simulink model "FSFB_PID_Controller"  (R2022a)
settings: Solver=VariableStepAuto  StartTime=0.0  StopTime=10.0  RelTol=1e-3
undefined symbols (not defined in the file): K1, K2, x_0
libraries: dspsigops x1
settings Model: Creator=domin  LastModifiedBy=domin
settings DataIOCC: SaveOutput=off  SaveTime=off
settings DebuggingCC: ModelReferenceExtraNoncontSigs=warning
settings GRTTargetCC: CombineOutputUpdateFcns=off  MatFileLogging=off

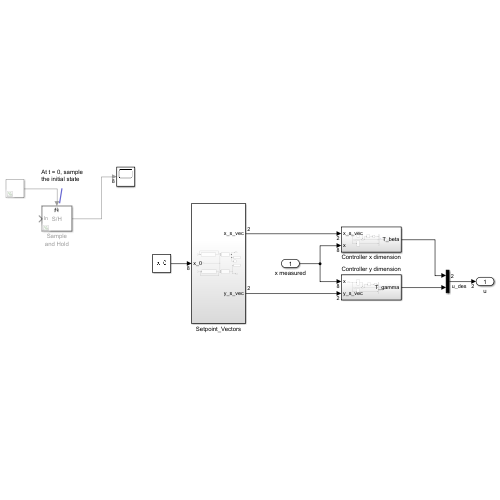
[thumbnail: Simulink's stored preview of the top-level diagram]
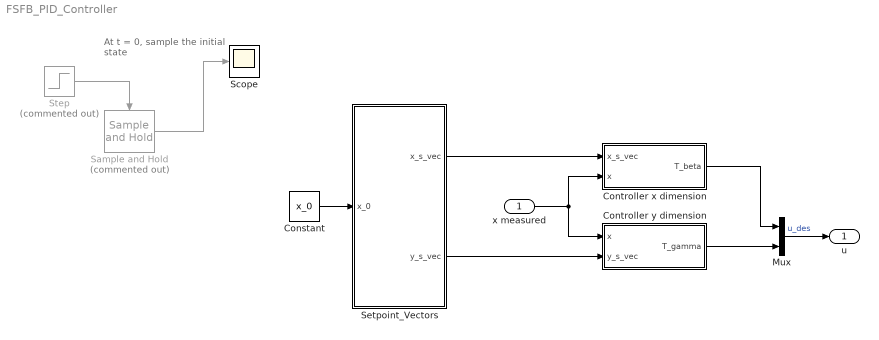
== system FSFB_PID_Controller ==
  note: At t = 0, sample the initial state
  x measured : Inport
  Constant : Constant  Value=x_0
  Controller x dimension : Subsystem
  Controller y dimension : Subsystem
  Mux : Mux  Inputs=2
  Sample and Hold : dspsigops/Sample and Hold  Commented=on  trig=Either edge  initCond=0  latchinput=off
  Scope : Scope
  Setpoint_Vectors : Subsystem
  Step : Step  Commented=on  Time=0.000001  SampleTime=0
  u : Outport
  wires:
  Controller x dimension/1(T_beta) -> Mux/1
  Mux/1 -> u/1  "u_des"
  x measured/1 -> Controller y dimension/1(x), Controller x dimension/2(x)
  Controller y dimension/1(T_gamma) -> Mux/2
  Setpoint_Vectors/1(x_s_vec) -> Controller x dimension/1(x_s_vec)
  Setpoint_Vectors/2(y_s_vec) -> Controller y dimension/2(y_s_vec)
  Step/1 -> Sample and Hold/Trigger
  Sample and Hold/1 -> Scope/1
  Constant/1 -> Setpoint_Vectors/1(x_0)

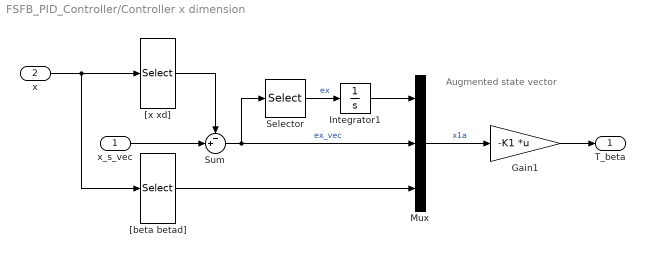
== system FSFB_PID_Controller/Controller x dimension ==
  note: Augmented state vector
  x_s_vec : Inport
  x : Inport  Port=2
  Gain1 : Gain  Gain=-K1  Multiplication=Matrix(K*u)
  Integrator1 : Integrator
  Mux : Mux  Inputs=3
  Selector : Selector  InputPortWidth=2  IndexOptions=Index vector (dialog)  Indices=[1 ]  OutputSizes=1
  Sum : Sum  Inputs=-+|
  "[beta betad]" : Selector  InputPortWidth=8  IndexOptions=Index vector (dialog)  Indices=[3,4]  OutputSizes=1
  "[x xd]" : Selector  InputPortWidth=8  IndexOptions=Index vector (dialog)  Indices=[1 2]  OutputSizes=1
  T_beta : Outport
  wires:
  "[beta betad]"/1 -> Mux/3
  Gain1/1 -> T_beta/1
  "[x xd]"/1 -> Sum/1
  Mux/1 -> Gain1/1  "x1a"
  Sum/1 -> Mux/2, Selector/1  "ex_vec"
  x_s_vec/1 -> Sum/2
  x/1 -> "[x xd]"/1, "[beta betad]"/1
  Selector/1 -> Integrator1/1  "ex"
  Integrator1/1 -> Mux/1

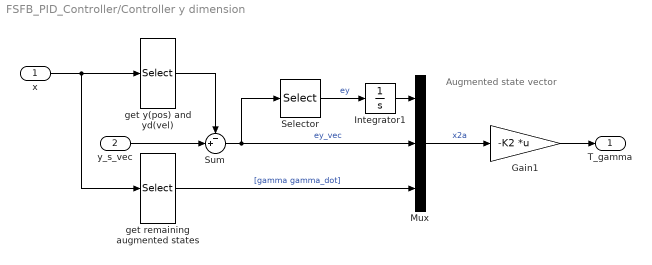
== system FSFB_PID_Controller/Controller y dimension ==
  note: Augmented state vector
  x : Inport
  y_s_vec : Inport  Port=2
  Gain1 : Gain  Gain=-K2  Multiplication=Matrix(K*u)
  Integrator1 : Integrator
  Mux : Mux  Inputs=3
  Selector : Selector  InputPortWidth=2  IndexOptions=Index vector (dialog)  Indices=[1 ]  OutputSizes=1
  Sum : Sum  Inputs=-+|
  get remaining augmented states : Selector  InputPortWidth=8  IndexOptions=Index vector (dialog)  Indices=[7 8]  OutputSizes=1
  get y(pos) and yd(vel) : Selector  InputPortWidth=8  IndexOptions=Index vector (dialog)  Indices=[5 6]  OutputSizes=1
  T_gamma : Outport
  wires:
  x/1 -> get y(pos) and yd(vel)/1, get remaining augmented states/1
  y_s_vec/1 -> Sum/2
  Selector/1 -> Integrator1/1  "ey"
  get y(pos) and yd(vel)/1 -> Sum/1
  Integrator1/1 -> Mux/1
  get remaining augmented states/1 -> Mux/3  "[gamma gamma_dot]"
  Sum/1 -> Mux/2, Selector/1  "ey_vec"
  Gain1/1 -> T_gamma/1
  Mux/1 -> Gain1/1  "x2a"

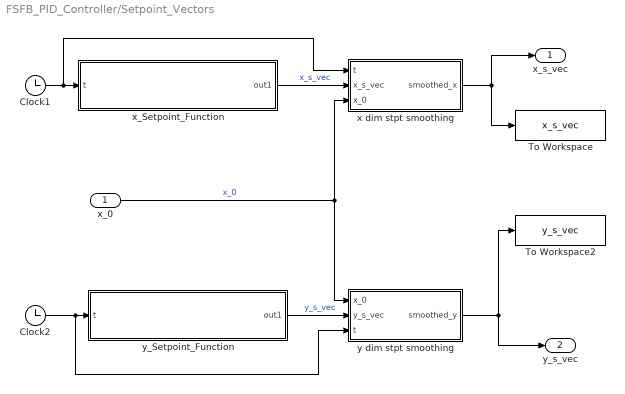
== system FSFB_PID_Controller/Setpoint_Vectors ==
  x_0 : Inport
  Clock1 : Clock
  Clock2 : Clock
  To Workspace : ToWorkspace  VariableName=x_s_vec  SampleTime=-1
  To Workspace2 : ToWorkspace  VariableName=y_s_vec  SampleTime=-1
  x dim stpt smoothing : MATLAB Function  TreatAsAtomicUnit=on
  x_Setpoint_Function : MATLAB Function  TreatAsAtomicUnit=on
  y dim stpt smoothing : MATLAB Function  TreatAsAtomicUnit=on
  y_Setpoint_Function : MATLAB Function  TreatAsAtomicUnit=on
  x_s_vec : Outport
  y_s_vec : Outport  Port=2
  wires:
  y dim stpt smoothing/1(smoothed_y) -> y_s_vec/1, To Workspace2/1
  y_Setpoint_Function/1(out1) -> y dim stpt smoothing/2(y_s_vec)  "y_s_vec"
  x dim stpt smoothing/1(smoothed_x) -> x_s_vec/1, To Workspace/1
  Clock1/1 -> x dim stpt smoothing/1(t), x_Setpoint_Function/1(t)
  Clock2/1 -> y dim stpt smoothing/3(t), y_Setpoint_Function/1(t)
  x_Setpoint_Function/1(out1) -> x dim stpt smoothing/2(x_s_vec)  "x_s_vec"
  x_0/1 -> x dim stpt smoothing/3(x_0), y dim stpt smoothing/1(x_0)  "x_0"

== matlab function FSFB_PID_Controller/Setpoint_Vectors/y dim stpt smoothing ==
  data: x_0 input size=8; y_s_vec input size=2; t input; smoothed_y output size=2; Tau parameter
function smoothed_y = fcn(x_0,y_s_vec,t, Tau)

smoothed_y = y_s_vec*(1-exp(-t/Tau)) + x_0(5:6)*exp(-t/Tau);

== matlab function FSFB_PID_Controller/Setpoint_Vectors/x_Setpoint_Function ==
  data: t input; out1 output
function out1 = x_s_vec(t)
%#codegen

%    This function was generated by the Symbolic Math Toolbox version 9.1.
%    05-Dec-2022 16:43:54

out1 = [-3.0./2.0e+1;0.0];

== matlab function FSFB_PID_Controller/Setpoint_Vectors/y_Setpoint_Function ==
  data: t input; out1 output
function out1 = y_s_vec(t)
%#codegen

%    This function was generated by the Symbolic Math Toolbox version 9.1.
%    05-Dec-2022 16:43:54

out1 = [-3.0./2.0e+1;0.0];

== matlab function FSFB_PID_Controller/Setpoint_Vectors/x dim stpt smoothing ==
  data: t input; x_s_vec input size=2; smoothed_x output size=2; Tau parameter; x_0 input size=8
function smoothed_x = fcn(t,x_s_vec, Tau, x_0)

smoothed_x = x_s_vec*(1-exp(-t/Tau)) + x_0(1:2)*exp(-t/Tau);
